simulink model "HANcoder_E407_TTA_Controller_v4_5"  (R2018b)
settings: Solver=FixedStepDiscrete  StartTime=0.0  StopTime=1  FixedStep=0.01  RelTol=1e-3
PreLoadFcn:
  | librarySetup
  | eval([bdroot,'_startup']) %Calling [modelName]_startup.m
values from neighbouring files (symbols this model uses):
  Backup_Board = 0    [HANcoder_E407_TTA_Controller_v3_5_startup.m]    (also in HANcoder_E407_TTA_Controller_v4_6_startup.m; HANcoder_E407_TTA_Controller_v4_7_startup.m; HANcoder_E407_TTA_Controller_v4_startup.m)
  basic_cycle_duration_bc0 = TM_Reset_Board   + COMP_duration    (= 212)    [HANcoder_E407_TTA_Controller_v3_5_startup.m]    (also in HANcoder_E407_TTA_Controller_v4_6_startup.m; HANcoder_E407_TTA_Controller_v4_7_startup.m; HANcoder_E407_TTA_Controller_v4_startup.m)
  basic_cycle_duration_bc1 = TM_Reset_Var_bc1 + COMP_duration    (= 288)    [HANcoder_E407_TTA_Controller_v3_5_startup.m]    (also in HANcoder_E407_TTA_Controller_v4_6_startup.m = 332; HANcoder_E407_TTA_Controller_v4_7_startup.m = 372; HANcoder_E407_TTA_Controller_v4_startup.m = 332)
  comm_delay_estimation1 = round(comm_delay_measured1*hardware_granularity/frequency_IRQ)    [HANcoder_E407_TTA_Controller_v3_5_startup.m]    (also in HANcoder_E407_TTA_Controller_v4_6_startup.m; HANcoder_E407_TTA_Controller_v4_7_startup.m; HANcoder_E407_TTA_Controller_v4_startup.m)
  comm_delay_estimation2 = round(comm_delay_measured2*hardware_granularity/frequency_IRQ)    [HANcoder_E407_TTA_Controller_v3_5_startup.m]    (also in HANcoder_E407_TTA_Controller_v4_6_startup.m; HANcoder_E407_TTA_Controller_v4_7_startup.m; HANcoder_E407_TTA_Controller_v4_startup.m)
  COMM_Period = 40    [HANcoder_E407_TTA_Controller_v3_5_startup.m]    (also in HANcoder_E407_TTA_Controller_v4_6_startup.m; HANcoder_E407_TTA_Controller_v4_7_startup.m; HANcoder_E407_TTA_Controller_v4_startup.m)
  COMM_Phase1 = Simulink.Parameter    [HANcoder_E407_TTA_Controller_v3_5_startup.m]    (also in HANcoder_E407_TTA_Controller_v4_6_startup.m; HANcoder_E407_TTA_Controller_v4_7_startup.m; HANcoder_E407_TTA_Controller_v4_startup.m)
  COMM_Phase2 = Simulink.Parameter    [HANcoder_E407_TTA_Controller_v3_5_startup.m]    (also in HANcoder_E407_TTA_Controller_v4_6_startup.m; HANcoder_E407_TTA_Controller_v4_7_startup.m; HANcoder_E407_TTA_Controller_v4_startup.m)
  COMM_Phase_init1 = Simulink.Parameter    [HANcoder_E407_TTA_Controller_v3_5_startup.m]    (also in HANcoder_E407_TTA_Controller_v4_6_startup.m; HANcoder_E407_TTA_Controller_v4_7_startup.m; HANcoder_E407_TTA_Controller_v4_startup.m)
  COMM_Phase_init2 = Simulink.Parameter    [HANcoder_E407_TTA_Controller_v3_5_startup.m]    (also in HANcoder_E407_TTA_Controller_v4_6_startup.m; HANcoder_E407_TTA_Controller_v4_7_startup.m; HANcoder_E407_TTA_Controller_v4_startup.m)
  COMP_duration = 4    [HANcoder_E407_TTA_Controller_v3_5_startup.m]    (also in HANcoder_E407_TTA_Controller_v4_6_startup.m; HANcoder_E407_TTA_Controller_v4_7_startup.m; HANcoder_E407_TTA_Controller_v4_startup.m)
  Controller1_Board = 1    [HANcoder_E407_TTA_Controller_v3_5_startup.m]    (also in HANcoder_E407_TTA_Controller_v4_6_startup.m; HANcoder_E407_TTA_Controller_v4_7_startup.m; HANcoder_E407_TTA_Controller_v4_startup.m)
  Controller2_Board = 2    [HANcoder_E407_TTA_Controller_v3_5_startup.m]    (also in HANcoder_E407_TTA_Controller_v4_6_startup.m; HANcoder_E407_TTA_Controller_v4_7_startup.m; HANcoder_E407_TTA_Controller_v4_startup.m)
  Controller3_Board = 3    [HANcoder_E407_TTA_Controller_v3_5_startup.m]    (also in HANcoder_E407_TTA_Controller_v4_6_startup.m; HANcoder_E407_TTA_Controller_v4_7_startup.m; HANcoder_E407_TTA_Controller_v4_startup.m)
  delta_a_set = Simulink.Parameter    [HANcoder_E407_TTA_Controller_v3_5_startup.m]    (also in HANcoder_E407_TTA_Controller_v4_6_startup.m; HANcoder_E407_TTA_Controller_v4_7_startup.m; HANcoder_E407_TTA_Controller_v4_startup.m)
  delta_f_set = Simulink.Parameter    [HANcoder_E407_TTA_Controller_v3_5_startup.m]    (also in HANcoder_E407_TTA_Controller_v4_6_startup.m; HANcoder_E407_TTA_Controller_v4_7_startup.m; HANcoder_E407_TTA_Controller_v4_startup.m)
  delta_max = 1    [HANcoder_E407_TTA_Controller_v3_5_startup.m]    (also in HANcoder_E407_TTA_Controller_v4_6_startup.m; HANcoder_E407_TTA_Controller_v4_7_startup.m; HANcoder_E407_TTA_Controller_v4_startup.m)
  delta_min = -1    [HANcoder_E407_TTA_Controller_v3_5_startup.m]    (also in HANcoder_E407_TTA_Controller_v4_6_startup.m; HANcoder_E407_TTA_Controller_v4_7_startup.m; HANcoder_E407_TTA_Controller_v4_startup.m)
  delta_precision = 6    [HANcoder_E407_TTA_Controller_v3_5_startup.m]    (also in HANcoder_E407_TTA_Controller_v4_6_startup.m; HANcoder_E407_TTA_Controller_v4_7_startup.m; HANcoder_E407_TTA_Controller_v4_startup.m)
  e_width = 0.1    [HANcoder_E407_TTA_Controller_v3_5_startup.m]    (also in HANcoder_E407_TTA_Controller_v4_6_startup.m; HANcoder_E407_TTA_Controller_v4_7_startup.m; HANcoder_E407_TTA_Controller_v4_startup.m)
  frequency_IRQ = 100    [HANcoder_E407_2xCAN_TEST_startup.m]    (also in HANcoder_E407_TTA_Controller_v3_5_startup.m; HANcoder_E407_TTA_Controller_v4_6_startup.m; HANcoder_E407_TTA_Controller_v4_7_startup.m; HANcoder_E407_TTA_Controller_v4_startup.m)
  HANtuneOverride = Simulink.Parameter    [HANcoder_E407_2xCAN_TEST_startup.m]    (also in HANcoder_E407_TTA_Controller_v3_5_startup.m; HANcoder_E407_TTA_Controller_v4_6_startup.m; HANcoder_E407_TTA_Controller_v4_7_startup.m; HANcoder_E407_TTA_Controller_v4_startup.m)
  hardware_granularity = 1000000    [HANcoder_E407_2xCAN_TEST_startup.m]    (also in HANcoder_E407_TTA_Controller_v3_5_startup.m; HANcoder_E407_TTA_Controller_v4_6_startup.m; HANcoder_E407_TTA_Controller_v4_7_startup.m; HANcoder_E407_TTA_Controller_v4_startup.m)
  I_a = 2.25    [HANcoder_E407_TTA_Controller_v3_5_startup.m]    (also in HANcoder_E407_TTA_Controller_v4_6_startup.m; HANcoder_E407_TTA_Controller_v4_7_startup.m; HANcoder_E407_TTA_Controller_v4_startup.m)
  I_f = 2.25    [HANcoder_E407_TTA_Controller_v3_5_startup.m]    (also in HANcoder_E407_TTA_Controller_v4_6_startup.m; HANcoder_E407_TTA_Controller_v4_7_startup.m; HANcoder_E407_TTA_Controller_v4_startup.m)
  idle_time_init = basic_cycle_duration_bc0 + basic_cycle_duration_bc1    (= 500)    [HANcoder_E407_TTA_Controller_v3_5_startup.m]    (also in HANcoder_E407_TTA_Controller_v4_6_startup.m = 544; HANcoder_E407_TTA_Controller_v4_7_startup.m = 584; HANcoder_E407_TTA_Controller_v4_startup.m = 544)
  Input_Gen_Board = 4    [HANcoder_E407_TTA_Controller_v3_5_startup.m]    (also in HANcoder_E407_TTA_Controller_v4_6_startup.m; HANcoder_E407_TTA_Controller_v4_7_startup.m; HANcoder_E407_TTA_Controller_v4_startup.m)
  LA_Clock_Gr = 1    [HANcoder_E407_TTA_Controller_v3_5_startup.m]    (also in HANcoder_E407_TTA_Controller_v4_6_startup.m; HANcoder_E407_TTA_Controller_v4_7_startup.m; HANcoder_E407_TTA_Controller_v4_startup.m)
  LA_COMM_dly = 1    [HANcoder_E407_TTA_Controller_v3_5_startup.m]    (also in HANcoder_E407_TTA_Controller_v4_6_startup.m; HANcoder_E407_TTA_Controller_v4_7_startup.m; HANcoder_E407_TTA_Controller_v4_startup.m)
  LA_COMM_Err = 1    [HANcoder_E407_TTA_Controller_v3_5_startup.m]    (also in HANcoder_E407_TTA_Controller_v4_6_startup.m; HANcoder_E407_TTA_Controller_v4_7_startup.m; HANcoder_E407_TTA_Controller_v4_startup.m)
  LA_E_Desync = 1    [HANcoder_E407_TTA_Controller_v3_5_startup.m]    (also in HANcoder_E407_TTA_Controller_v4_6_startup.m; HANcoder_E407_TTA_Controller_v4_7_startup.m; HANcoder_E407_TTA_Controller_v4_startup.m)
  LA_MEX_Flag = 1    [HANcoder_E407_TTA_Controller_v3_5_startup.m]    (also in HANcoder_E407_TTA_Controller_v4_6_startup.m; HANcoder_E407_TTA_Controller_v4_7_startup.m; HANcoder_E407_TTA_Controller_v4_startup.m)
  LA_Task_Act = 1    [HANcoder_E407_TTA_Controller_v3_5_startup.m]    (also in HANcoder_E407_TTA_Controller_v4_6_startup.m; HANcoder_E407_TTA_Controller_v4_7_startup.m; HANcoder_E407_TTA_Controller_v4_startup.m)
  m_v = 100.0    (= 100)    [HANcoder_E407_TTA_Controller_v3_5_startup.m]    (also in HANcoder_E407_TTA_Controller_v4_6_startup.m; HANcoder_E407_TTA_Controller_v4_7_startup.m; HANcoder_E407_TTA_Controller_v4_startup.m)
  Master_Role = 1    [HANcoder_E407_TTA_Controller_v3_5_startup.m]    (also in HANcoder_E407_TTA_Controller_v4_6_startup.m; HANcoder_E407_TTA_Controller_v4_7_startup.m; HANcoder_E407_TTA_Controller_v4_startup.m)
  matrix_cycle_duration = basic_cycle_duration_bc0 + basic_cycle_duration_bc1    (= 500)    [HANcoder_E407_TTA_Controller_v3_5_startup.m]    (also in HANcoder_E407_TTA_Controller_v4_6_startup.m = 544; HANcoder_E407_TTA_Controller_v4_7_startup.m = 584; HANcoder_E407_TTA_Controller_v4_startup.m = 544)
  matrix_rows = 2    [HANcoder_E407_TTA_Controller_v3_5_startup.m]    (also in HANcoder_E407_TTA_Controller_v4_6_startup.m; HANcoder_E407_TTA_Controller_v4_7_startup.m; HANcoder_E407_TTA_Controller_v4_startup.m)
  max_desync = 15    [HANcoder_E407_TTA_Controller_v3_5_startup.m]    (also in HANcoder_E407_TTA_Controller_v4_6_startup.m; HANcoder_E407_TTA_Controller_v4_7_startup.m = 30; HANcoder_E407_TTA_Controller_v4_startup.m)
  max_num_msgs_CAN1 = 2^Tx_bit_number-1    (= 7)    [HANcoder_E407_TTA_Controller_v3_5_startup.m]    (also in HANcoder_E407_TTA_Controller_v4_6_startup.m = 15; HANcoder_E407_TTA_Controller_v4_7_startup.m = 15; HANcoder_E407_TTA_Controller_v4_startup.m)
  max_num_msgs_CAN2 = max_num_msgs_CAN1    (= 7)    [HANcoder_E407_TTA_Controller_v3_5_startup.m]    (also in HANcoder_E407_TTA_Controller_v4_6_startup.m = 15; HANcoder_E407_TTA_Controller_v4_7_startup.m = 15; HANcoder_E407_TTA_Controller_v4_startup.m)
  min_desync = (-1)*max_desync    (= -15)    [HANcoder_E407_TTA_Controller_v3_5_startup.m]    (also in HANcoder_E407_TTA_Controller_v4_6_startup.m; HANcoder_E407_TTA_Controller_v4_7_startup.m = -30; HANcoder_E407_TTA_Controller_v4_startup.m)
  OutControl1_ID = 23    [HANcoder_E407_TTA_Controller_v3_5_startup.m]    (also in HANcoder_E407_TTA_Controller_v4_6_startup.m; HANcoder_E407_TTA_Controller_v4_7_startup.m; HANcoder_E407_TTA_Controller_v4_startup.m)
  OutControl2_ID = 24    [HANcoder_E407_TTA_Controller_v3_5_startup.m]    (also in HANcoder_E407_TTA_Controller_v4_6_startup.m; HANcoder_E407_TTA_Controller_v4_7_startup.m; HANcoder_E407_TTA_Controller_v4_startup.m)
  OutEmulator_ID = 25    [HANcoder_E407_TTA_Controller_v3_5_startup.m]    (also in HANcoder_E407_TTA_Controller_v4_6_startup.m = 26; HANcoder_E407_TTA_Controller_v4_7_startup.m = 26; HANcoder_E407_TTA_Controller_v4_startup.m)
  OutMaster_ID = 25    [HANcoder_E407_TTA_Controller_v4_6_startup.m]    (also in HANcoder_E407_TTA_Controller_v4_7_startup.m; HANcoder_E407_TTA_Controller_v4_startup.m = 26)
  R_al = 0.10    (= 0.1)    [HANcoder_E407_TTA_Controller_v3_5_startup.m]    (also in HANcoder_E407_TTA_Controller_v4_6_startup.m; HANcoder_E407_TTA_Controller_v4_7_startup.m; HANcoder_E407_TTA_Controller_v4_startup.m)
  R_ar = 0.10    (= 0.1)    [HANcoder_E407_TTA_Controller_v3_5_startup.m]    (also in HANcoder_E407_TTA_Controller_v4_6_startup.m; HANcoder_E407_TTA_Controller_v4_7_startup.m; HANcoder_E407_TTA_Controller_v4_startup.m)
  R_fl = 0.10    (= 0.1)    [HANcoder_E407_TTA_Controller_v3_5_startup.m]    (also in HANcoder_E407_TTA_Controller_v4_6_startup.m; HANcoder_E407_TTA_Controller_v4_7_startup.m; HANcoder_E407_TTA_Controller_v4_startup.m)
  R_fr = 0.10    (= 0.1)    [HANcoder_E407_TTA_Controller_v3_5_startup.m]    (also in HANcoder_E407_TTA_Controller_v4_6_startup.m; HANcoder_E407_TTA_Controller_v4_7_startup.m; HANcoder_E407_TTA_Controller_v4_startup.m)
  script_run = Simulink.Parameter    [HANcoder_E407_TTA_Controller_v3_5_startup.m]    (also in HANcoder_E407_TTA_Controller_v4_6_startup.m; HANcoder_E407_TTA_Controller_v4_7_startup.m; HANcoder_E407_TTA_Controller_v4_startup.m)
  SensorValues_ID = 22    [HANcoder_E407_TTA_Controller_v3_5_startup.m]    (also in HANcoder_E407_TTA_Controller_v4_6_startup.m; HANcoder_E407_TTA_Controller_v4_7_startup.m; HANcoder_E407_TTA_Controller_v4_startup.m)
  SetValues_ID = 21    [HANcoder_E407_TTA_Controller_v3_5_startup.m]    (also in HANcoder_E407_TTA_Controller_v4_6_startup.m; HANcoder_E407_TTA_Controller_v4_7_startup.m; HANcoder_E407_TTA_Controller_v4_startup.m)
  Slave_Role = 2    [HANcoder_E407_TTA_Controller_v3_5_startup.m]    (also in HANcoder_E407_TTA_Controller_v4_6_startup.m; HANcoder_E407_TTA_Controller_v4_7_startup.m; HANcoder_E407_TTA_Controller_v4_startup.m)
  speed_k_d = Simulink.Parameter    [HANcoder_E407_TTA_Controller_v3_5_startup.m]    (also in HANcoder_E407_TTA_Controller_v4_6_startup.m; HANcoder_E407_TTA_Controller_v4_7_startup.m; HANcoder_E407_TTA_Controller_v4_startup.m)
  speed_k_i = Simulink.Parameter    [HANcoder_E407_TTA_Controller_v3_5_startup.m]    (also in HANcoder_E407_TTA_Controller_v4_6_startup.m; HANcoder_E407_TTA_Controller_v4_7_startup.m; HANcoder_E407_TTA_Controller_v4_startup.m)
  speed_k_p = Simulink.Parameter    [HANcoder_E407_TTA_Controller_v3_5_startup.m]    (also in HANcoder_E407_TTA_Controller_v4_6_startup.m; HANcoder_E407_TTA_Controller_v4_7_startup.m; HANcoder_E407_TTA_Controller_v4_startup.m)
  speed_max = 10    [HANcoder_E407_TTA_Controller_v3_5_startup.m]    (also in HANcoder_E407_TTA_Controller_v4_6_startup.m; HANcoder_E407_TTA_Controller_v4_7_startup.m; HANcoder_E407_TTA_Controller_v4_startup.m)
  speed_min = -10    [HANcoder_E407_TTA_Controller_v3_5_startup.m]    (also in HANcoder_E407_TTA_Controller_v4_6_startup.m; HANcoder_E407_TTA_Controller_v4_7_startup.m; HANcoder_E407_TTA_Controller_v4_startup.m)
  speed_precision = 3    [HANcoder_E407_TTA_Controller_v3_5_startup.m]    (also in HANcoder_E407_TTA_Controller_v4_6_startup.m; HANcoder_E407_TTA_Controller_v4_7_startup.m; HANcoder_E407_TTA_Controller_v4_startup.m)
  Sync_ID = 1    [HANcoder_E407_TTA_Controller_v3_5_startup.m]    (also in HANcoder_E407_TTA_Controller_v4_6_startup.m; HANcoder_E407_TTA_Controller_v4_7_startup.m; HANcoder_E407_TTA_Controller_v4_startup.m)
  tau_max = 5    [HANcoder_E407_TTA_Controller_v3_5_startup.m]    (also in HANcoder_E407_TTA_Controller_v4_6_startup.m; HANcoder_E407_TTA_Controller_v4_7_startup.m; HANcoder_E407_TTA_Controller_v4_startup.m)
  tau_min = -5    [HANcoder_E407_TTA_Controller_v3_5_startup.m]    (also in HANcoder_E407_TTA_Controller_v4_6_startup.m; HANcoder_E407_TTA_Controller_v4_7_startup.m; HANcoder_E407_TTA_Controller_v4_startup.m)
  tau_range = abs(tau_max) + abs(tau_min)    [HANcoder_E407_TTA_Controller_v3_5_startup.m]    (also in HANcoder_E407_TTA_Controller_v4_6_startup.m; HANcoder_E407_TTA_Controller_v4_7_startup.m; HANcoder_E407_TTA_Controller_v4_startup.m)
  theta_max = (speed_max/R_fr)*matrix_cycle_duration*frequency_IRQ/hardware_granularity    (= 5)    [HANcoder_E407_TTA_Controller_v3_5_startup.m]    (also in HANcoder_E407_TTA_Controller_v4_6_startup.m = 5.44; HANcoder_E407_TTA_Controller_v4_7_startup.m = 5.84; HANcoder_E407_TTA_Controller_v4_startup.m = 5.44)
  theta_min = (-1)*theta_max    (= -5)    [HANcoder_E407_TTA_Controller_v3_5_startup.m]    (also in HANcoder_E407_TTA_Controller_v4_6_startup.m = -5.44; HANcoder_E407_TTA_Controller_v4_7_startup.m = -5.84; HANcoder_E407_TTA_Controller_v4_startup.m = -5.44)
  theta_precision = 7-(fix(log2(theta_max))+1)    [HANcoder_E407_TTA_Controller_v3_5_startup.m]    (also in HANcoder_E407_TTA_Controller_v4_6_startup.m; HANcoder_E407_TTA_Controller_v4_7_startup.m; HANcoder_E407_TTA_Controller_v4_startup.m)
  Tl_a = 0.6    [HANcoder_E407_TTA_Controller_v3_5_startup.m]    (also in HANcoder_E407_TTA_Controller_v4_6_startup.m; HANcoder_E407_TTA_Controller_v4_7_startup.m; HANcoder_E407_TTA_Controller_v4_startup.m)
  Tl_f = 0.6    [HANcoder_E407_TTA_Controller_v3_5_startup.m]    (also in HANcoder_E407_TTA_Controller_v4_6_startup.m; HANcoder_E407_TTA_Controller_v4_7_startup.m; HANcoder_E407_TTA_Controller_v4_startup.m)
  TM_Check_Output_Control1 = TM_COMM_Output_Control1 + COMM_duration    (= 188)    [HANcoder_E407_TTA_Controller_v3_5_startup.m]    (also in HANcoder_E407_TTA_Controller_v4_6_startup.m; HANcoder_E407_TTA_Controller_v4_7_startup.m; HANcoder_E407_TTA_Controller_v4_startup.m)
  TM_Check_Output_Control2 = TM_COMM_Output_Control2 + COMM_duration    (= 232)    [HANcoder_E407_TTA_Controller_v3_5_startup.m]    (also in HANcoder_E407_TTA_Controller_v4_6_startup.m; HANcoder_E407_TTA_Controller_v4_7_startup.m; HANcoder_E407_TTA_Controller_v4_startup.m)
  TM_Check_Output_Emulator = TM_COMM_Output_Emulator + COMM_duration    (= 280)    [HANcoder_E407_TTA_Controller_v3_5_startup.m]    (also in HANcoder_E407_TTA_Controller_v4_6_startup.m = 320; HANcoder_E407_TTA_Controller_v4_7_startup.m = 360; HANcoder_E407_TTA_Controller_v4_startup.m = 320)
  TM_Check_Output_Emulator_2 = TM_Check_Output_Emulator + 2    (= 282)    [HANcoder_E407_TTA_Controller_v3_5_startup.m]    (also in HANcoder_E407_TTA_Controller_v4_6_startup.m = 322; HANcoder_E407_TTA_Controller_v4_7_startup.m = 362; HANcoder_E407_TTA_Controller_v4_startup.m = 322)
  TM_Check_Output_Emulator_3 = TM_Check_Output_Emulator_2 + 2    (= 324)    [HANcoder_E407_TTA_Controller_v4_6_startup.m]    (also in HANcoder_E407_TTA_Controller_v4_7_startup.m = 364; HANcoder_E407_TTA_Controller_v4_startup.m)
  TM_Check_Sensor_Values = TM_COMM_Sensor_Values + COMM_duration    (= 132)    [HANcoder_E407_TTA_Controller_v3_5_startup.m]    (also in HANcoder_E407_TTA_Controller_v4_6_startup.m; HANcoder_E407_TTA_Controller_v4_7_startup.m; HANcoder_E407_TTA_Controller_v4_startup.m)
  TM_Check_Sensor_Values_2 = TM_Check_Sensor_Values + 2    (= 134)    [HANcoder_E407_TTA_Controller_v3_5_startup.m]    (also in HANcoder_E407_TTA_Controller_v4_6_startup.m; HANcoder_E407_TTA_Controller_v4_7_startup.m; HANcoder_E407_TTA_Controller_v4_startup.m)
  TM_Check_Set_Values = TM_COMM_Set_Values + COMM_duration    (= 88)    [HANcoder_E407_TTA_Controller_v3_5_startup.m]    (also in HANcoder_E407_TTA_Controller_v4_6_startup.m; HANcoder_E407_TTA_Controller_v4_7_startup.m; HANcoder_E407_TTA_Controller_v4_startup.m)
  TM_Check_Set_Values_2 = TM_Check_Set_Values + 2    (= 90)    [HANcoder_E407_TTA_Controller_v3_5_startup.m]    (also in HANcoder_E407_TTA_Controller_v4_6_startup.m; HANcoder_E407_TTA_Controller_v4_7_startup.m; HANcoder_E407_TTA_Controller_v4_startup.m)
  TM_Check_Sync = TM_COMM_Sync   + COMM_duration    (= 40)    [HANcoder_E407_TTA_Controller_v3_5_startup.m]    (also in HANcoder_E407_TTA_Controller_v4_6_startup.m; HANcoder_E407_TTA_Controller_v4_7_startup.m; HANcoder_E407_TTA_Controller_v4_startup.m)
  TM_Check_TOuts = TM_Count_Vote3 + COMP_duration    (= 196)    [HANcoder_E407_TTA_Controller_v3_5_startup.m]    (also in HANcoder_E407_TTA_Controller_v4_6_startup.m; HANcoder_E407_TTA_Controller_v4_7_startup.m; HANcoder_E407_TTA_Controller_v4_startup.m)
  TM_Check_Vote1 = TM_COMM_Vote1  + COMM_duration    (= 92)    [HANcoder_E407_TTA_Controller_v3_5_startup.m]    (also in HANcoder_E407_TTA_Controller_v4_6_startup.m; HANcoder_E407_TTA_Controller_v4_7_startup.m; HANcoder_E407_TTA_Controller_v4_startup.m)
  TM_Check_Vote2 = TM_COMM_Vote2  + COMM_duration    (= 140)    [HANcoder_E407_TTA_Controller_v3_5_startup.m]    (also in HANcoder_E407_TTA_Controller_v4_6_startup.m; HANcoder_E407_TTA_Controller_v4_7_startup.m; HANcoder_E407_TTA_Controller_v4_startup.m)
  TM_Check_Vote2_2 = TM_Check_Vote2 + 2    (= 142)    [HANcoder_E407_TTA_Controller_v3_5_startup.m]    (also in HANcoder_E407_TTA_Controller_v4_6_startup.m; HANcoder_E407_TTA_Controller_v4_7_startup.m; HANcoder_E407_TTA_Controller_v4_startup.m)
  TM_Check_Vote3 = TM_COMM_Vote3  + COMM_duration    (= 188)    [HANcoder_E407_TTA_Controller_v3_5_startup.m]    (also in HANcoder_E407_TTA_Controller_v4_6_startup.m; HANcoder_E407_TTA_Controller_v4_7_startup.m; HANcoder_E407_TTA_Controller_v4_startup.m)
  TM_COMM_Output_Control1 = TM_Velocity + COMP_duration    (= 148)    [HANcoder_E407_TTA_Controller_v3_5_startup.m]    (also in HANcoder_E407_TTA_Controller_v4_6_startup.m; HANcoder_E407_TTA_Controller_v4_7_startup.m; HANcoder_E407_TTA_Controller_v4_startup.m)
  TM_COMM_Output_Control2 = TM_Check_Output_Control1 + COMP_duration    (= 192)    [HANcoder_E407_TTA_Controller_v3_5_startup.m]    (also in HANcoder_E407_TTA_Controller_v4_6_startup.m; HANcoder_E407_TTA_Controller_v4_7_startup.m; HANcoder_E407_TTA_Controller_v4_startup.m)
  TM_COMM_Output_Emulator = TM_TMR + COMP_duration    (= 240)    [HANcoder_E407_TTA_Controller_v3_5_startup.m]    (also in HANcoder_E407_TTA_Controller_v4_6_startup.m = 280; HANcoder_E407_TTA_Controller_v4_7_startup.m = 320; HANcoder_E407_TTA_Controller_v4_startup.m = 280)
  TM_COMM_Output_Master = TM_Check_Output_Control2 + COMM_duration    (= 272)    [HANcoder_E407_TTA_Controller_v4_6_startup.m]    (also in HANcoder_E407_TTA_Controller_v4_7_startup.m; HANcoder_E407_TTA_Controller_v4_startup.m)
  TM_COMM_Sensor_Values = TM_Check_Set_Values + COMP_duration    (= 92)    [HANcoder_E407_TTA_Controller_v3_5_startup.m]    (also in HANcoder_E407_TTA_Controller_v4_6_startup.m; HANcoder_E407_TTA_Controller_v4_7_startup.m; HANcoder_E407_TTA_Controller_v4_startup.m)
  TM_COMM_Set_Values = TM_Update_LT + COMP_duration    (= 48)    [HANcoder_E407_TTA_Controller_v3_5_startup.m]    (also in HANcoder_E407_TTA_Controller_v4_6_startup.m; HANcoder_E407_TTA_Controller_v4_7_startup.m; HANcoder_E407_TTA_Controller_v4_startup.m)
  TM_COMM_Sync = basic_cycle_start    (= 0)    [HANcoder_E407_TTA_Controller_v3_5_startup.m]    (also in HANcoder_E407_TTA_Controller_v4_6_startup.m; HANcoder_E407_TTA_Controller_v4_7_startup.m; HANcoder_E407_TTA_Controller_v4_startup.m)
  TM_COMM_Vote1 = TM_Vote_Dec    + COMP_duration    (= 52)    [HANcoder_E407_TTA_Controller_v3_5_startup.m]    (also in HANcoder_E407_TTA_Controller_v4_6_startup.m; HANcoder_E407_TTA_Controller_v4_7_startup.m; HANcoder_E407_TTA_Controller_v4_startup.m)
  TM_COMM_Vote2 = TM_Count_Vote1 + COMP_duration    (= 100)    [HANcoder_E407_TTA_Controller_v3_5_startup.m]    (also in HANcoder_E407_TTA_Controller_v4_6_startup.m; HANcoder_E407_TTA_Controller_v4_7_startup.m; HANcoder_E407_TTA_Controller_v4_startup.m)
  TM_COMM_Vote3 = TM_Count_Vote2 + COMP_duration    (= 148)    [HANcoder_E407_TTA_Controller_v3_5_startup.m]    (also in HANcoder_E407_TTA_Controller_v4_6_startup.m; HANcoder_E407_TTA_Controller_v4_7_startup.m; HANcoder_E407_TTA_Controller_v4_startup.m)
  TM_Count_Vote1 = TM_Check_Vote1 + COMP_duration    (= 96)    [HANcoder_E407_TTA_Controller_v3_5_startup.m]    (also in HANcoder_E407_TTA_Controller_v4_6_startup.m; HANcoder_E407_TTA_Controller_v4_7_startup.m; HANcoder_E407_TTA_Controller_v4_startup.m)
  TM_Count_Vote2 = TM_Check_Vote2 + COMP_duration    (= 144)    [HANcoder_E407_TTA_Controller_v3_5_startup.m]    (also in HANcoder_E407_TTA_Controller_v4_6_startup.m; HANcoder_E407_TTA_Controller_v4_7_startup.m; HANcoder_E407_TTA_Controller_v4_startup.m)
  TM_Count_Vote3 = TM_Check_Vote3 + COMP_duration    (= 192)    [HANcoder_E407_TTA_Controller_v3_5_startup.m]    (also in HANcoder_E407_TTA_Controller_v4_6_startup.m; HANcoder_E407_TTA_Controller_v4_7_startup.m; HANcoder_E407_TTA_Controller_v4_startup.m)
  TM_Data_bc0 = TM_COMM_Sync    (= 0)    [HANcoder_E407_TTA_Controller_v3_5_startup.m]    (also in HANcoder_E407_TTA_Controller_v4_6_startup.m; HANcoder_E407_TTA_Controller_v4_7_startup.m; HANcoder_E407_TTA_Controller_v4_startup.m)
  TM_Data_bc1 = TM_Data_bc0(1:4)    [HANcoder_E407_TTA_Controller_v3_5_startup.m]    (also in HANcoder_E407_TTA_Controller_v4_6_startup.m; HANcoder_E407_TTA_Controller_v4_7_startup.m; HANcoder_E407_TTA_Controller_v4_startup.m)
  TM_New_Master = TM_Check_TOuts + COMP_duration    (= 200)    [HANcoder_E407_TTA_Controller_v3_5_startup.m]    (also in HANcoder_E407_TTA_Controller_v4_6_startup.m; HANcoder_E407_TTA_Controller_v4_7_startup.m; HANcoder_E407_TTA_Controller_v4_startup.m)
  TM_Reset_Board = TM_Reset_Var   + COMP_duration    (= 208)    [HANcoder_E407_TTA_Controller_v3_5_startup.m]    (also in HANcoder_E407_TTA_Controller_v4_6_startup.m; HANcoder_E407_TTA_Controller_v4_7_startup.m; HANcoder_E407_TTA_Controller_v4_startup.m)
  TM_Reset_Var = TM_New_Master  + COMP_duration    (= 204)    [HANcoder_E407_TTA_Controller_v3_5_startup.m]    (also in HANcoder_E407_TTA_Controller_v4_6_startup.m; HANcoder_E407_TTA_Controller_v4_7_startup.m; HANcoder_E407_TTA_Controller_v4_startup.m)
  TM_Reset_Var_bc1 = TM_Check_Output_Emulator + COMP_duration    (= 284)    [HANcoder_E407_TTA_Controller_v3_5_startup.m]    (also in HANcoder_E407_TTA_Controller_v4_6_startup.m = 328; HANcoder_E407_TTA_Controller_v4_7_startup.m = 368; HANcoder_E407_TTA_Controller_v4_startup.m = 328)
  TM_Reset_Var_bc1_2 = TM_Reset_Var_bc1 + 2    (= 286)    [HANcoder_E407_TTA_Controller_v3_5_startup.m]    (also in HANcoder_E407_TTA_Controller_v4_6_startup.m = 330; HANcoder_E407_TTA_Controller_v4_7_startup.m = 370; HANcoder_E407_TTA_Controller_v4_startup.m = 330)
  TM_Steer = TM_Check_Sensor_Values + COMP_duration    (= 136)    [HANcoder_E407_TTA_Controller_v3_5_startup.m]    (also in HANcoder_E407_TTA_Controller_v4_6_startup.m; HANcoder_E407_TTA_Controller_v4_7_startup.m; HANcoder_E407_TTA_Controller_v4_startup.m)
  TM_TMR = TM_Check_Output_Control2 + COMP_duration    (= 236)    [HANcoder_E407_TTA_Controller_v3_5_startup.m]    (also in HANcoder_E407_TTA_Controller_v4_6_startup.m = 276; HANcoder_E407_TTA_Controller_v4_7_startup.m = 316; HANcoder_E407_TTA_Controller_v4_startup.m = 276)
  TM_TMR_2 = TM_TMR + 1    (= 237)    [HANcoder_E407_TTA_Controller_v3_5_startup.m]    (also in HANcoder_E407_TTA_Controller_v4_6_startup.m = 277; HANcoder_E407_TTA_Controller_v4_7_startup.m = 317; HANcoder_E407_TTA_Controller_v4_startup.m = 277)
  TM_TMR_3 = TM_TMR + 3    (= 239)    [HANcoder_E407_TTA_Controller_v3_5_startup.m]    (also in HANcoder_E407_TTA_Controller_v4_6_startup.m = 279; HANcoder_E407_TTA_Controller_v4_7_startup.m = 319; HANcoder_E407_TTA_Controller_v4_startup.m = 279)
  TM_Torque = TM_Steer + COMP_duration    (= 140)    [HANcoder_E407_TTA_Controller_v3_5_startup.m]    (also in HANcoder_E407_TTA_Controller_v4_6_startup.m; HANcoder_E407_TTA_Controller_v4_7_startup.m; HANcoder_E407_TTA_Controller_v4_startup.m)
  TM_Type_bc0 = COMM    (= 0)    [HANcoder_E407_TTA_Controller_v3_5_startup.m]    (also in HANcoder_E407_TTA_Controller_v4_6_startup.m; HANcoder_E407_TTA_Controller_v4_7_startup.m; HANcoder_E407_TTA_Controller_v4_startup.m)
  TM_Type_bc1 = TM_Type_bc0(1:4)    [HANcoder_E407_TTA_Controller_v3_5_startup.m]    (also in HANcoder_E407_TTA_Controller_v4_6_startup.m; HANcoder_E407_TTA_Controller_v4_7_startup.m; HANcoder_E407_TTA_Controller_v4_startup.m)
  TM_Update_LT = TM_Check_Sync  + COMP_duration    (= 44)    [HANcoder_E407_TTA_Controller_v3_5_startup.m]    (also in HANcoder_E407_TTA_Controller_v4_6_startup.m; HANcoder_E407_TTA_Controller_v4_7_startup.m; HANcoder_E407_TTA_Controller_v4_startup.m)
  TM_Update_LT_2 = TM_Update_LT   + 2    (= 46)    [HANcoder_E407_TTA_Controller_v3_5_startup.m]    (also in HANcoder_E407_TTA_Controller_v4_6_startup.m; HANcoder_E407_TTA_Controller_v4_7_startup.m; HANcoder_E407_TTA_Controller_v4_startup.m)
  TM_Velocity = TM_Torque + COMP_duration    (= 144)    [HANcoder_E407_TTA_Controller_v3_5_startup.m]    (also in HANcoder_E407_TTA_Controller_v4_6_startup.m; HANcoder_E407_TTA_Controller_v4_7_startup.m; HANcoder_E407_TTA_Controller_v4_startup.m)
  TM_Vote_Dec = TM_Update_LT   + COMP_duration    (= 48)    [HANcoder_E407_TTA_Controller_v3_5_startup.m]    (also in HANcoder_E407_TTA_Controller_v4_6_startup.m; HANcoder_E407_TTA_Controller_v4_7_startup.m; HANcoder_E407_TTA_Controller_v4_startup.m)
  TM_Vote_Dec_2 = TM_Vote_Dec    + 2    (= 50)    [HANcoder_E407_TTA_Controller_v3_5_startup.m]    (also in HANcoder_E407_TTA_Controller_v4_6_startup.m; HANcoder_E407_TTA_Controller_v4_7_startup.m; HANcoder_E407_TTA_Controller_v4_startup.m)
  torque_a_k_d = Simulink.Parameter    [HANcoder_E407_TTA_Controller_v3_5_startup.m]    (also in HANcoder_E407_TTA_Controller_v4_6_startup.m; HANcoder_E407_TTA_Controller_v4_7_startup.m; HANcoder_E407_TTA_Controller_v4_startup.m)
  torque_a_k_i = Simulink.Parameter    [HANcoder_E407_TTA_Controller_v3_5_startup.m]    (also in HANcoder_E407_TTA_Controller_v4_6_startup.m; HANcoder_E407_TTA_Controller_v4_7_startup.m; HANcoder_E407_TTA_Controller_v4_startup.m)
  torque_a_k_p = Simulink.Parameter    [HANcoder_E407_TTA_Controller_v3_5_startup.m]    (also in HANcoder_E407_TTA_Controller_v4_6_startup.m; HANcoder_E407_TTA_Controller_v4_7_startup.m; HANcoder_E407_TTA_Controller_v4_startup.m)
  torque_f_k_d = Simulink.Parameter    [HANcoder_E407_TTA_Controller_v3_5_startup.m]    (also in HANcoder_E407_TTA_Controller_v4_6_startup.m; HANcoder_E407_TTA_Controller_v4_7_startup.m; HANcoder_E407_TTA_Controller_v4_startup.m)
  torque_f_k_i = Simulink.Parameter    [HANcoder_E407_TTA_Controller_v3_5_startup.m]    (also in HANcoder_E407_TTA_Controller_v4_6_startup.m; HANcoder_E407_TTA_Controller_v4_7_startup.m; HANcoder_E407_TTA_Controller_v4_startup.m)
  ... (+7 more)
undefined symbols (not defined in the file or in its folder): A0, A1, A2, A3, A4, CON2, CON3, CON4, D10, D12, D13, D2, D3, D8, D9
libraries: hdlsllib x467, HANcoder_STM32_Target x30, simulink x3, simulink_extras x1
(part 20 of 80)

== system HANcoder_E407_TTA_Controller_v4_5/HANcoder STM32 Target - E407-STM32 algorithm/TTA CAN System/TTA System/Matrix Cycle Manager/Controller Matrix Cycle/controller basic cycle 0/COMP Task - Vote2 Count ==
  note: Reception condition
  note: BC 0 TW6
      | Vote 1 count
  note: The own vote is stored in the second buffer
      | (Msg_Value_Data at COMM)
  Time Mark : Inport
  Enable : EnablePort
  AND : Logic  Inputs=3  IconShape=distinctive  AllPortsSameDT=off  OutDataTypeStr=boolean
  Bus Selector : BusSelector  OutputSignals=Buffer_2
  Constant4 : Constant  Value=2
  Data Store Read : DataStoreRead  DataStoreName=Local_Ticks
  Data Store Read1 : DataStoreRead  DataStoreName=Board_ID
  Data Store Read4 : DataStoreRead  DataStoreName=Msg_Rx
  Data Store Read5 : DataStoreRead  DataStoreName=new_msg_Rx
  Equal : RelationalOperator  Operator===  OutDataTypeStr=boolean  RndMeth=Simplest
  Equal2 : RelationalOperator  Operator=~=  OutDataTypeStr=boolean  RndMeth=Simplest
  Vote Count 2 : Subsystem
  wires:
  Bus Selector/1 -> Vote Count 2/1(Msg_Data)  "<Buffer_2>"
  Data Store Read4/1 -> Bus Selector/1
  Data Store Read5/1 -> AND/2
  Constant4/1 -> Equal2/2
  Data Store Read1/1 -> Equal2/1
  Equal2/1 -> AND/3
  Time Mark/1 -> Equal/2
  Data Store Read/1 -> Equal/1
  Equal/1 -> AND/1
  AND/1 -> Vote Count 2/Enable

== system HANcoder_E407_TTA_Controller_v4_5/HANcoder STM32 Target - E407-STM32 algorithm/TTA CAN System/TTA System/Matrix Cycle Manager/Controller Matrix Cycle/controller basic cycle 0/COMP Task - Vote2 check ==
  note: Reception condition
  note: Message information
  Time_Mark : Inport
  Enable : EnablePort
  AND : Logic  IconShape=distinctive  AllPortsSameDT=off  OutDataTypeStr=boolean
  AND1 : Logic  IconShape=distinctive  AllPortsSameDT=off  OutDataTypeStr=boolean
  Constant1 : Constant  Value=Controller2_Board
  Constant2 : Constant  Value=Controller2_Board
  Data Store Read : DataStoreRead  DataStoreName=Msg_Rx_CAN1
  Data Store Read1 : DataStoreRead  DataStoreName=New_Msg_Ready_CAN1
  Data Store Read2 : DataStoreRead  DataStoreName=New_Msg_Ready_CAN2
  Data Store Read21 : DataStoreRead  DataStoreName=Board_ID
  Data Store Read3 : DataStoreRead  DataStoreName=Msg_Rx_CAN2
  Data Store Read4 : DataStoreRead  DataStoreName=Local_Ticks
  Equal : RelationalOperator  Operator===  OutDataTypeStr=boolean  RndMeth=Simplest
  Equal6 : RelationalOperator  Operator=~=  OutDataTypeStr=boolean  RndMeth=Simplest
  NOT : Logic  Operator=NOT  IconShape=distinctive  AllPortsSameDT=off  OutDataTypeStr=boolean
  Process_Messages : Subsystem  Priority=20
  Reset Tx msg counter : Subsystem  TreatAsAtomicUnit=on
  wires:
  Constant2/1 -> Equal6/2
  Data Store Read21/1 -> Equal6/1
  Equal6/1 -> NOT/1, AND/2
  [First_Tick_TAG] -> AND/1
  [First_Tick_TAG] -> AND1/1
  Equal/1 -> [First_Tick_TAG]
  NOT/1 -> AND1/2
  AND1/1 -> Reset Tx msg counter/Enable
  AND/1 -> Process_Messages/Enable
  Data Store Read4/1 -> Equal/1
  Data Store Read3/1 -> Process_Messages/4(Rx_Msg_CAN2)
  Data Store Read/1 -> Process_Messages/3(Rx_msg_CAN1)
  Data Store Read2/1 -> Process_Messages/2(new_CAN2_msg)
  Data Store Read1/1 -> Process_Messages/1(new_CAN1_msg)
  Constant1/1 -> Process_Messages/5(expected_board_id)
  Time_Mark/1 -> Equal/2

== system HANcoder_E407_TTA_Controller_v4_5/HANcoder STM32 Target - E407-STM32 algorithm/TTA CAN System/TTA System/Matrix Cycle Manager/Controller Matrix Cycle/controller basic cycle 0/COMP Task - Vote3 Count ==
  note: The own vote is stored in the second buffer
      | (Msg_Value_Data at COMM)
  note: BC 0 TW6
      | Vote 1 count
  note: Reception condition
  Time Mark : Inport
  Enable : EnablePort
  AND : Logic  Inputs=3  IconShape=distinctive  AllPortsSameDT=off  OutDataTypeStr=boolean
  Bus Selector : BusSelector  OutputSignals=Buffer_2
  Constant4 : Constant  Value=3
  Data Store Read : DataStoreRead  DataStoreName=Local_Ticks
  Data Store Read1 : DataStoreRead  DataStoreName=Board_ID
  Data Store Read4 : DataStoreRead  DataStoreName=Msg_Rx
  Data Store Read5 : DataStoreRead  DataStoreName=new_msg_Rx
  Equal : RelationalOperator  Operator===  OutDataTypeStr=boolean  RndMeth=Simplest
  Equal2 : RelationalOperator  Operator=~=  OutDataTypeStr=boolean  RndMeth=Simplest
  Vote Count 3 : Subsystem
  wires:
  AND/1 -> Vote Count 3/Enable
  Equal/1 -> AND/1
  Data Store Read/1 -> Equal/1
  Time Mark/1 -> Equal/2
  Equal2/1 -> AND/3
  Data Store Read1/1 -> Equal2/1
  Constant4/1 -> Equal2/2
  Data Store Read5/1 -> AND/2
  Data Store Read4/1 -> Bus Selector/1
  Bus Selector/1 -> Vote Count 3/1(Msg_Data)  "<Buffer_2>"

== system HANcoder_E407_TTA_Controller_v4_5/HANcoder STM32 Target - E407-STM32 algorithm/TTA CAN System/TTA System/Matrix Cycle Manager/Controller Matrix Cycle/controller basic cycle 0/COMP Task - Vote3 check ==
  note: Message information
  note: Reception condition
  Time_Mark : Inport
  Enable : EnablePort
  AND : Logic  IconShape=distinctive  AllPortsSameDT=off  OutDataTypeStr=boolean
  AND1 : Logic  IconShape=distinctive  AllPortsSameDT=off  OutDataTypeStr=boolean
  Constant1 : Constant  Value=Controller3_Board
  Constant2 : Constant  Value=Controller3_Board
  Data Store Read : DataStoreRead  DataStoreName=Msg_Rx_CAN1
  Data Store Read1 : DataStoreRead  DataStoreName=New_Msg_Ready_CAN1
  Data Store Read2 : DataStoreRead  DataStoreName=New_Msg_Ready_CAN2
  Data Store Read21 : DataStoreRead  DataStoreName=Board_ID
  Data Store Read3 : DataStoreRead  DataStoreName=Msg_Rx_CAN2
  Data Store Read4 : DataStoreRead  DataStoreName=Local_Ticks
  Equal : RelationalOperator  Operator===  OutDataTypeStr=boolean  RndMeth=Simplest
  Equal6 : RelationalOperator  Operator=~=  OutDataTypeStr=boolean  RndMeth=Simplest
  NOT : Logic  Operator=NOT  IconShape=distinctive  AllPortsSameDT=off  OutDataTypeStr=boolean
  Process_Messages : Subsystem  Priority=20
  Reset Tx msg counter : Subsystem  TreatAsAtomicUnit=on
  wires:
  Time_Mark/1 -> Equal/2
  Constant1/1 -> Process_Messages/5(expected_board_id)
  Data Store Read1/1 -> Process_Messages/1(new_CAN1_msg)
  Data Store Read2/1 -> Process_Messages/2(new_CAN2_msg)
  Data Store Read/1 -> Process_Messages/3(Rx_msg_CAN1)
  Data Store Read3/1 -> Process_Messages/4(Rx_Msg_CAN2)
  Data Store Read4/1 -> Equal/1
  AND/1 -> Process_Messages/Enable
  AND1/1 -> Reset Tx msg counter/Enable
  NOT/1 -> AND1/2
  Equal/1 -> [First_Tick_TAG]
  [First_Tick_TAG] -> AND1/1
  [First_Tick_TAG] -> AND/1
  Equal6/1 -> AND/2, NOT/1
  Data Store Read21/1 -> Equal6/1
  Constant2/1 -> Equal6/2

== system HANcoder_E407_TTA_Controller_v4_5/HANcoder STM32 Target - E407-STM32 algorithm/TTA CAN System/TTA System/Matrix Cycle Manager/Controller Matrix Cycle/controller basic cycle 1/COMM Task - Output Control1 ==
  note: Tx condition
  note: The COMM task actions are different if the board must transmit (Tx) or receive (Rx)
  Time Mark : Inport
  Enable : EnablePort
  Constant70 : Constant  Value=OutControl1_ID
  NOT : Logic  Operator=NOT  IconShape=distinctive  AllPortsSameDT=off  OutDataTypeStr=boolean
  OutputControl1 Tx condition : Subsystem
  Reception substasks : Subsystem  TreatAsAtomicUnit=on
  Transmission subtasks1 : Subsystem  TreatAsAtomicUnit=on
  Send CAN1 : Outport  OutputWhenDisabled=reset  InitialOutput=0
  Receive CAN1 : Outport  Port=2  OutputWhenDisabled=reset  InitialOutput=0
  Send CAN2 : Outport  Port=3  OutputWhenDisabled=reset  InitialOutput=0
  Receive CAN2 : Outport  Port=4  OutputWhenDisabled=reset  InitialOutput=0
  wires:
  [Time_Mark_TAG] -> Reception substasks/1(Time_Mark)
  [Time_Mark_TAG] -> Transmission subtasks1/1(Time_Mark)
  Time Mark/1 -> [Time_Mark_TAG]
  [Msg_ID_TAG] -> Reception substasks/2(RX_ID)
  [Msg_ID_TAG] -> Transmission subtasks1/2(TX_ID)
  Constant70/1 -> [Msg_ID_TAG]
  Transmission subtasks1/2(Send CAN2) -> Send CAN2/1
  Transmission subtasks1/1(Send CAN1) -> Send CAN1/1
  Reception substasks/2(Receive CAN2) -> Receive CAN2/1
  Reception substasks/1(Receive CAN1) -> Receive CAN1/1
  NOT/1 -> Reception substasks/Enable
  OutputControl1 Tx condition/1(Tx_Board_Out1) -> Transmission subtasks1/Enable, NOT/1

== system HANcoder_E407_TTA_Controller_v4_5/HANcoder STM32 Target - E407-STM32 algorithm/TTA CAN System/TTA System/Matrix Cycle Manager/Controller Matrix Cycle/controller basic cycle 1/COMM Task - Output Control2 ==
  note: The COMM task actions are different if the board must transmit (Tx) or receive (Rx)
  note: Tx condition
  Time Mark : Inport
  Enable : EnablePort
  Constant86 : Constant  Value=OutControl2_ID
  NOT : Logic  Operator=NOT  IconShape=distinctive  AllPortsSameDT=off  OutDataTypeStr=boolean
  OutputControl2 Tx condition : Subsystem
  Reception substasks : Subsystem  TreatAsAtomicUnit=on
  Transmission subtasks : Subsystem  TreatAsAtomicUnit=on
  Send CAN1 : Outport  OutputWhenDisabled=reset  InitialOutput=0
  Receive CAN1 : Outport  Port=2  OutputWhenDisabled=reset  InitialOutput=0
  Send CAN2 : Outport  Port=3  OutputWhenDisabled=reset  InitialOutput=0
  Receive CAN2 : Outport  Port=4  OutputWhenDisabled=reset  InitialOutput=0
  wires:
  OutputControl2 Tx condition/1(Tx_Board_Out2) -> Transmission subtasks/Enable, NOT/1
  NOT/1 -> Reception substasks/Enable
  Reception substasks/1(Receive CAN1) -> Receive CAN1/1
  Reception substasks/2(Receive CAN2) -> Receive CAN2/1
  Transmission subtasks/1(Send CAN1) -> Send CAN1/1
  Transmission subtasks/2(Send CAN2) -> Send CAN2/1
  Constant86/1 -> [Msg_ID_TAG]
  [Msg_ID_TAG] -> Transmission subtasks/2(TX_ID)
  [Msg_ID_TAG] -> Reception substasks/2(RX_ID)
  Time Mark/1 -> [Time_Mark_TAG]
  [Time_Mark_TAG] -> Transmission subtasks/1(Time_Mark)
  [Time_Mark_TAG] -> Reception substasks/1(Time_Mark)

== system HANcoder_E407_TTA_Controller_v4_5/HANcoder STM32 Target - E407-STM32 algorithm/TTA CAN System/TTA System/Matrix Cycle Manager/Controller Matrix Cycle/controller basic cycle 1/COMM Task - Output Control3 ==
  note: The COMM task actions are different if the board must transmit (Tx) or receive (Rx)
  note: Tx condition
  Time Mark : Inport
  Enable : EnablePort
  Constant86 : Constant  Value=OutMaster_ID
  NOT : Logic  Operator=NOT  IconShape=distinctive  AllPortsSameDT=off  OutDataTypeStr=boolean
  OutputControl2 Tx condition : Subsystem
  Reception substasks : Subsystem  TreatAsAtomicUnit=on
  Transmission subtasks : Subsystem  TreatAsAtomicUnit=on
  Send CAN1 : Outport  OutputWhenDisabled=reset  InitialOutput=0
  Receive CAN1 : Outport  Port=2  OutputWhenDisabled=reset  InitialOutput=0
  Send CAN2 : Outport  Port=3  OutputWhenDisabled=reset  InitialOutput=0
  Receive CAN2 : Outport  Port=4  OutputWhenDisabled=reset  InitialOutput=0
  wires:
  OutputControl2 Tx condition/1(Tx_Board_Out2) -> Transmission subtasks/Enable, NOT/1
  NOT/1 -> Reception substasks/Enable
  Reception substasks/1(Receive CAN1) -> Receive CAN1/1
  Reception substasks/2(Receive CAN2) -> Receive CAN2/1
  Transmission subtasks/1(Send CAN1) -> Send CAN1/1
  Transmission subtasks/2(Send CAN2) -> Send CAN2/1
  Constant86/1 -> [Msg_ID_TAG]
  [Msg_ID_TAG] -> Transmission subtasks/2(TX_ID)
  [Msg_ID_TAG] -> Reception substasks/2(RX_ID)
  Time Mark/1 -> [Time_Mark_TAG]
  [Time_Mark_TAG] -> Transmission subtasks/1(Time_Mark)
  [Time_Mark_TAG] -> Reception substasks/1(Time_Mark)

== system HANcoder_E407_TTA_Controller_v4_5/HANcoder STM32 Target - E407-STM32 algorithm/TTA CAN System/TTA System/Matrix Cycle Manager/Controller Matrix Cycle/controller basic cycle 1/COMM Task - Output Emulator ==
  note: Tx condition
  note: The COMM task actions are different if the board must transmit (Tx) or receive (Rx)
  Time Mark : Inport
  Enable : EnablePort
  Constant95 : Constant  Value=OutEmulator_ID
  Constant98 : Constant  Value=Master_Role
  Data Store Read31 : DataStoreRead  DataStoreName=Role_ID
  Equal17 : RelationalOperator  Operator===  OutDataTypeStr=boolean  RndMeth=Simplest
  NOT : Logic  Operator=NOT  IconShape=distinctive  AllPortsSameDT=off  OutDataTypeStr=boolean
  Reception substasks : Subsystem  TreatAsAtomicUnit=on
  Transmission subtasks : Subsystem  TreatAsAtomicUnit=on
  Send CAN1 : Outport  OutputWhenDisabled=reset  InitialOutput=0
  Receive CAN1 : Outport  Port=2  OutputWhenDisabled=reset  InitialOutput=0
  Send CAN2 : Outport  Port=3  OutputWhenDisabled=reset  InitialOutput=0
  Receive CAN2 : Outport  Port=4  OutputWhenDisabled=reset  InitialOutput=0
  wires:
  [Time_Mark_TAG] -> Reception substasks/1(Time_Mark)
  [Time_Mark_TAG] -> Transmission subtasks/1(Time_Mark)
  Time Mark/1 -> [Time_Mark_TAG]
  [Msg_ID_TAG] -> Reception substasks/2(RX_ID)
  [Msg_ID_TAG] -> Transmission subtasks/2(TX_ID)
  Constant95/1 -> [Msg_ID_TAG]
  Transmission subtasks/2(Send CAN2) -> Send CAN2/1
  Transmission subtasks/1(Send CAN1) -> Send CAN1/1
  Reception substasks/2(Receive CAN2) -> Receive CAN2/1
  Reception substasks/1(Receive CAN1) -> Receive CAN1/1
  NOT/1 -> Reception substasks/Enable
  Equal17/1 -> Transmission subtasks/Enable, NOT/1
  Data Store Read31/1 -> Equal17/1
  Constant98/1 -> Equal17/2

== system HANcoder_E407_TTA_Controller_v4_5/HANcoder STM32 Target - E407-STM32 algorithm/TTA CAN System/TTA System/Matrix Cycle Manager/Controller Matrix Cycle/controller basic cycle 1/COMM Task - Sensor_Values ==
  note: The COMM task actions are different if the board must transmit (Tx) or receive (Rx)
  note: Tx condition
  Time Mark : Inport
  Enable : EnablePort
  Constant66 : Constant  Value=Vehicle_Em_Board
  Constant70 : Constant  Value=SensorValues_ID
  Data Store Read26 : DataStoreRead  DataStoreName=Board_ID
  Equal12 : RelationalOperator  Operator===  OutDataTypeStr=boolean  RndMeth=Simplest
  NOT : Logic  Operator=NOT  IconShape=distinctive  AllPortsSameDT=off  OutDataTypeStr=boolean
  Reception substasks : Subsystem  TreatAsAtomicUnit=on
  Transmission subtasks : Subsystem  TreatAsAtomicUnit=on
  Send CAN1 : Outport  OutputWhenDisabled=reset  InitialOutput=0
  Receive CAN1 : Outport  Port=2  OutputWhenDisabled=reset  InitialOutput=0
  Send CAN2 : Outport  Port=3  OutputWhenDisabled=reset  InitialOutput=0
  Receive CAN2 : Outport  Port=4  OutputWhenDisabled=reset  InitialOutput=0
  wires:
  Data Store Read26/1 -> Equal12/1
  Constant66/1 -> Equal12/2
  Equal12/1 -> Transmission subtasks/Enable, NOT/1
  NOT/1 -> Reception substasks/Enable
  Reception substasks/1(Receive CAN1) -> Receive CAN1/1
  Reception substasks/2(Receive CAN2) -> Receive CAN2/1
  Transmission subtasks/1(Send CAN1) -> Send CAN1/1
  Transmission subtasks/2(Send CAN2) -> Send CAN2/1
  Constant70/1 -> [Msg_ID_TAG]
  [Msg_ID_TAG] -> Transmission subtasks/2(TX_ID)
  [Msg_ID_TAG] -> Reception substasks/2(RX_ID)
  Time Mark/1 -> [Time_Mark_TAG]
  [Time_Mark_TAG] -> Transmission subtasks/1(Time_Mark)
  [Time_Mark_TAG] -> Reception substasks/1(Time_Mark)

== system HANcoder_E407_TTA_Controller_v4_5/HANcoder STM32 Target - E407-STM32 algorithm/TTA CAN System/TTA System/Matrix Cycle Manager/Controller Matrix Cycle/controller basic cycle 1/COMM Task - Set_Values ==
  note: Tx condition
  note: The COMM task actions are different if the board must transmit (Tx) or receive (Rx)
  Time Mark : Inport
  Enable : EnablePort
  Constant55 : Constant  Value=Input_Gen_Board
  Constant59 : Constant  Value=SetValues_ID
  Data Store Read26 : DataStoreRead  DataStoreName=Board_ID
  Equal12 : RelationalOperator  Operator===  OutDataTypeStr=boolean  RndMeth=Simplest
  NOT : Logic  Operator=NOT  IconShape=distinctive  AllPortsSameDT=off  OutDataTypeStr=boolean
  Reception substasks : Subsystem  TreatAsAtomicUnit=on
  Transmission subtasks : Subsystem  TreatAsAtomicUnit=on
  Send CAN1 : Outport  OutputWhenDisabled=reset  InitialOutput=0
  Receive CAN1 : Outport  Port=2  OutputWhenDisabled=reset  InitialOutput=0
  Send CAN2 : Outport  Port=3  OutputWhenDisabled=reset  InitialOutput=0
  Receive CAN2 : Outport  Port=4  OutputWhenDisabled=reset  InitialOutput=0
  wires:
  [Time_Mark_TAG] -> Reception substasks/1(Time_Mark)
  [Time_Mark_TAG] -> Transmission subtasks/1(Time_Mark)
  Time Mark/1 -> [Time_Mark_TAG]
  [Msg_ID_TAG] -> Reception substasks/2(RX_ID)
  [Msg_ID_TAG] -> Transmission subtasks/2(TX_ID)
  Constant59/1 -> [Msg_ID_TAG]
  Transmission subtasks/2(Send CAN2) -> Send CAN2/1
  Transmission subtasks/1(Send CAN1) -> Send CAN1/1
  Reception substasks/2(Receive CAN2) -> Receive CAN2/1
  Reception substasks/1(Receive CAN1) -> Receive CAN1/1
  NOT/1 -> Reception substasks/Enable
  Equal12/1 -> Transmission subtasks/Enable, NOT/1
  Constant55/1 -> Equal12/2
  Data Store Read26/1 -> Equal12/1

== system HANcoder_E407_TTA_Controller_v4_5/HANcoder STM32 Target - E407-STM32 algorithm/TTA CAN System/TTA System/Matrix Cycle Manager/Controller Matrix Cycle/controller basic cycle 1/COMM Task - Sync bc 1 ==
  note: The COMM task actions are different if the board must transmit (Tx) or receive (Rx)
  note: Tx condition
  Time Mark : Inport
  Enable : EnablePort
  Constant : Constant  Value=Sync_ID
  Constant2 : Constant  Value=Master_Role
  Data Store Read1 : DataStoreRead  DataStoreName=Role_ID
  Equal1 : RelationalOperator  Operator===  OutDataTypeStr=boolean  RndMeth=Simplest
  NOT : Logic  Operator=NOT  IconShape=distinctive  AllPortsSameDT=off  OutDataTypeStr=boolean
  Reception substasks : Subsystem  TreatAsAtomicUnit=on
  Transmission subtasks1 : Subsystem  TreatAsAtomicUnit=on
  Send CAN1 : Outport  OutputWhenDisabled=reset  InitialOutput=0
  Receive CAN1 : Outport  Port=2  OutputWhenDisabled=reset  InitialOutput=0
  Send CAN2 : Outport  Port=3  OutputWhenDisabled=reset  InitialOutput=0
  Receive CAN2 : Outport  Port=4  OutputWhenDisabled=reset  InitialOutput=0
  wires:
  Constant2/1 -> Equal1/2
  Data Store Read1/1 -> Equal1/1
  Equal1/1 -> Transmission subtasks1/Enable, NOT/1
  NOT/1 -> Reception substasks/Enable
  Reception substasks/1(Receive CAN1) -> Receive CAN1/1
  Reception substasks/2(Receive CAN2) -> Receive CAN2/1
  Transmission subtasks1/1(Send CAN1) -> Send CAN1/1
  Transmission subtasks1/2(Send CAN2) -> Send CAN2/1
  Constant/1 -> [Msg_ID_TAG]
  [Msg_ID_TAG] -> Transmission subtasks1/2(TX_ID)
  [Msg_ID_TAG] -> Reception substasks/2(RX_ID)
  Time Mark/1 -> [Time_Mark_TAG]
  [Time_Mark_TAG] -> Transmission subtasks1/1(Time_Mark)
  [Time_Mark_TAG] -> Reception substasks/1(Time_Mark)

== system HANcoder_E407_TTA_Controller_v4_5/HANcoder STM32 Target - E407-STM32 algorithm/TTA CAN System/TTA System/Matrix Cycle Manager/Controller Matrix Cycle/controller basic cycle 1/COMP Task - Calculate Speed ==
  note: BC 1 TW 9
      | Calculate speed
  note: Make calculations if we got both inputs
  Time_Mark : Inport
  Enable : EnablePort
  AND : Logic  IconShape=distinctive  AllPortsSameDT=off  OutDataTypeStr=boolean
  Calculate speed : Subsystem  TreatAsAtomicUnit=on
  Data Store Read : DataStoreRead  DataStoreName=Local_Ticks
  Data Store Read1 : DataStoreRead  Priority=121  DataStoreName=Error_SensorValues_NotRX
  Data Store Read2 : DataStoreRead  Priority=120  DataStoreName=Error_SetValues_NotRX
  Equal : RelationalOperator  Operator===  OutDataTypeStr=boolean  RndMeth=Simplest
  NOT : Logic  Operator=NOT  IconShape=distinctive  AllPortsSameDT=off  OutDataTypeStr=boolean
  OR : Logic  Operator=OR  IconShape=distinctive  AllPortsSameDT=off  OutDataTypeStr=boolean
  wires:
  Data Store Read/1 -> Equal/1
  Time_Mark/1 -> Equal/2
  OR/1 -> NOT/1
  NOT/1 -> AND/2
  Data Store Read1/1 -> OR/2
  Data Store Read2/1 -> OR/1
  AND/1 -> Calculate speed/Enable
  Equal/1 -> AND/1

== system HANcoder_E407_TTA_Controller_v4_5/HANcoder STM32 Target - E407-STM32 algorithm/TTA CAN System/TTA System/Matrix Cycle Manager/Controller Matrix Cycle/controller basic cycle 1/COMP Task - Calculate Steer ==
  note: BC 1 TW 7
      | Calculate steering
  note: Make calculations if we got both inputs
  Time_Mark : Inport
  Enable : EnablePort
  AND : Logic  IconShape=distinctive  AllPortsSameDT=off  OutDataTypeStr=boolean
  Calculate steering : Subsystem  TreatAsAtomicUnit=on
  Data Store Read : DataStoreRead  DataStoreName=Local_Ticks
  Data Store Read1 : DataStoreRead  Priority=121  DataStoreName=Error_SensorValues_NotRX
  Data Store Read2 : DataStoreRead  Priority=120  DataStoreName=Error_SetValues_NotRX
  Equal : RelationalOperator  Operator===  OutDataTypeStr=boolean  RndMeth=Simplest
  NOT : Logic  Operator=NOT  IconShape=distinctive  AllPortsSameDT=off  OutDataTypeStr=boolean
  OR : Logic  Operator=OR  IconShape=distinctive  AllPortsSameDT=off  OutDataTypeStr=boolean
  wires:
  Data Store Read/1 -> Equal/1
  Time_Mark/1 -> Equal/2
  OR/1 -> NOT/1
  NOT/1 -> AND/2
  Data Store Read1/1 -> OR/2
  Data Store Read2/1 -> OR/1
  AND/1 -> Calculate steering/Enable
  Equal/1 -> AND/1
